simulink model "Vehicle"  (R2023b)
settings: Solver=VariableStepAuto  StartTime=0.0  StopTime=1000  RelTol=1e-3
values from neighbouring files (symbols this model uses):
  Area = 2.5    [paras_Vehicle.m]
  b = 0.1    [paras_Vehicle.m]
  Capacity = 5    [paras_Vehicle.m]
  Cd = 0.3    [paras_Vehicle.m]
  G_ratio = 10    [paras_Vehicle.m]
  J = 0.01    [paras_Vehicle.m]
  L = 0.5    [paras_Vehicle.m]
  m_car = 1000    [paras_Vehicle.m]
  R = 1    [paras_Vehicle.m]
  R_bat = 0.5    [paras_Vehicle.m]
  r_tire = 0.3    [paras_Vehicle.m]
  rho = 1.225    [paras_Vehicle.m]
settings Model: Creator=mdhel  LastModifiedBy=mdhel

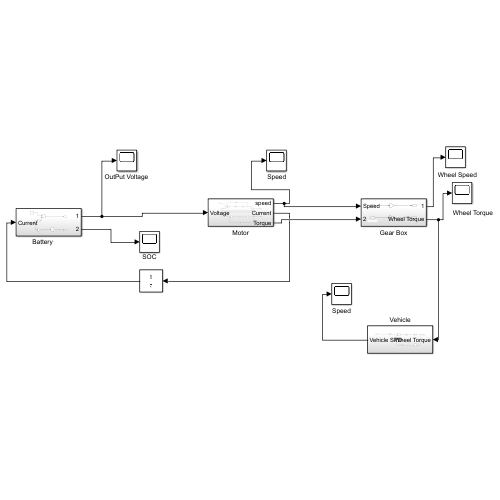
[thumbnail: Simulink's stored preview of the top-level diagram]
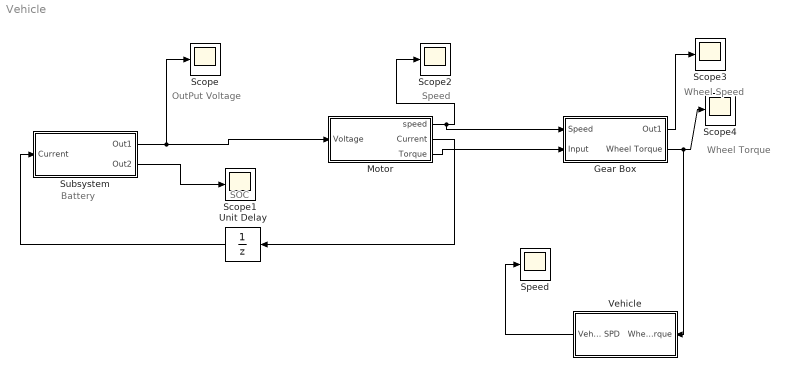
== system Vehicle ==
  note: Battery
  note: Wheel Speed
  note: OutPut Voltage
  note: Wheel Torque
  note: Speed
  note: SOC
  Gear Box : Subsystem
  Motor : Subsystem
  Scope{,1..4} (5 alike) : Scope
  Speed : Scope
  Subsystem : Subsystem
  Unit Delay : UnitDelay  SampleTime=-1  HasFrameUpgradeWarning=on
  Vehicle : Subsystem
  wires:
  Motor/3(Torque) -> Gear Box/2(Input)
  Gear Box/1(Out1) -> Scope3/1
  Gear Box/2(Wheel Torque) -> Vehicle/1(Wheel Torque), Scope4/1
  Subsystem/1(Out1) -> Motor/1(Voltage), Scope/1
  Subsystem/2(Out2) -> Scope1/1
  Unit Delay/1 -> Subsystem/1(Current)
  Motor/1(speed) -> Gear Box/1(Speed), Scope2/1
  Motor/2(Current) -> Unit Delay/1
  Vehicle/1(Vehicle SPD) -> Speed/1

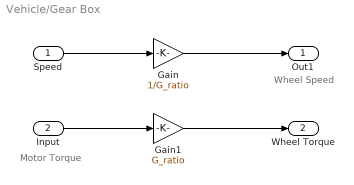
== system Vehicle/Gear Box ==
  note: Motor Torque
  note: Wheel Speed
  Speed : Inport
  Input : Inport  Port=2
  Gain : Gain  Gain=1/G_ratio
  Gain1 : Gain  Gain=G_ratio
  Out1 : Outport
  Wheel Torque : Outport  Port=2
  wires:
  Speed/1 -> Gain/1
  Gain/1 -> Out1/1
  Input/1 -> Gain1/1
  Gain1/1 -> Wheel Torque/1

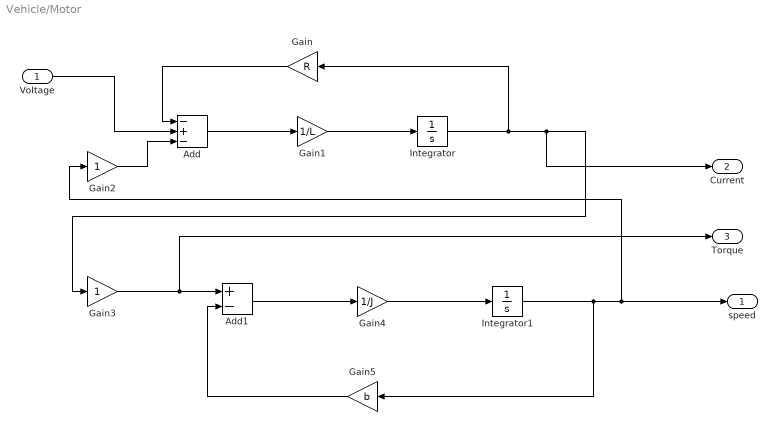
== system Vehicle/Motor ==
  Voltage : Inport
  Add : Sum  Inputs=-+-
  Add1 : Sum  Inputs=+-
  Gain : Gain  Gain=R
  Gain1 : Gain  Gain=1/L
  Gain2 : Gain
  Gain3 : Gain
  Gain4 : Gain  Gain=1/J
  Gain5 : Gain  Gain=b
  Integrator : Integrator
  Integrator1 : Integrator
  speed : Outport
  Current : Outport  Port=2
  Torque : Outport  Port=3
  wires:
  Voltage/1 -> Add/2
  Gain/1 -> Add/1
  Add/1 -> Gain1/1
  Gain1/1 -> Integrator/1
  Integrator/1 -> Gain/1, Current/1, Gain3/1
  Gain2/1 -> Add/3
  Gain3/1 -> Torque/1, Add1/1
  Add1/1 -> Gain4/1
  Gain4/1 -> Integrator1/1
  Integrator1/1 -> Gain5/1, Gain2/1, speed/1
  Gain5/1 -> Add1/2

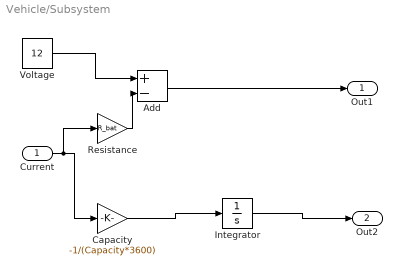
== system Vehicle/Subsystem ==
  Current : Inport
  Add : Sum  Inputs=+-
  Capacity : Gain  Gain=-1/(Capacity*3600)
  Integrator : Integrator  InitialCondition=1
  Resistance : Gain  Gain=R_bat
  Voltage : Constant  Value=12
  Out1 : Outport
  Out2 : Outport  Port=2
  wires:
  Voltage/1 -> Add/1
  Add/1 -> Out1/1
  Capacity/1 -> Integrator/1
  Integrator/1 -> Out2/1
  Current/1 -> Resistance/1, Capacity/1
  Resistance/1 -> Add/2

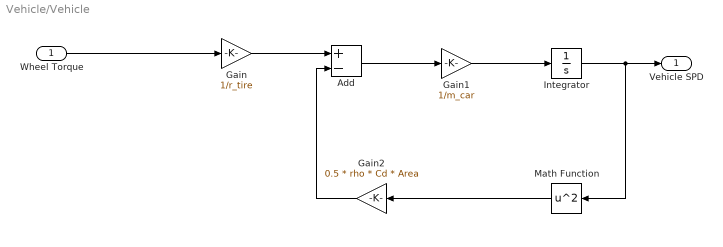
== system Vehicle/Vehicle ==
  Wheel Torque : Inport
  Add : Sum  Inputs=+-
  Gain : Gain  Gain=1/r_tire
  Gain1 : Gain  Gain=1/m_car
  Gain2 : Gain  Gain=0.5 * rho * Cd * Area
  Integrator : Integrator
  Math Function : Math  Operator=square
  Vehicle SPD : Outport
  wires:
  Wheel Torque/1 -> Gain/1
  Gain/1 -> Add/1
  Add/1 -> Gain1/1
  Gain1/1 -> Integrator/1
  Integrator/1 -> Math Function/1, Vehicle SPD/1
  Gain2/1 -> Add/2
  Math Function/1 -> Gain2/1
